simulink subsystem "Tractive_Motor_Ring_Single_Motor_subsys"  (R2020a)
settings: Solver=VariableStepAuto  StartTime=0.0  StopTime=10.0  RelTol=1e-3
undefined symbols (not defined in the file): DiscIntNeverNeededParam, magnitude, TMR
libraries: simulink x3
settings Model: Creator=Harjot  LastModifiedBy=Harjot

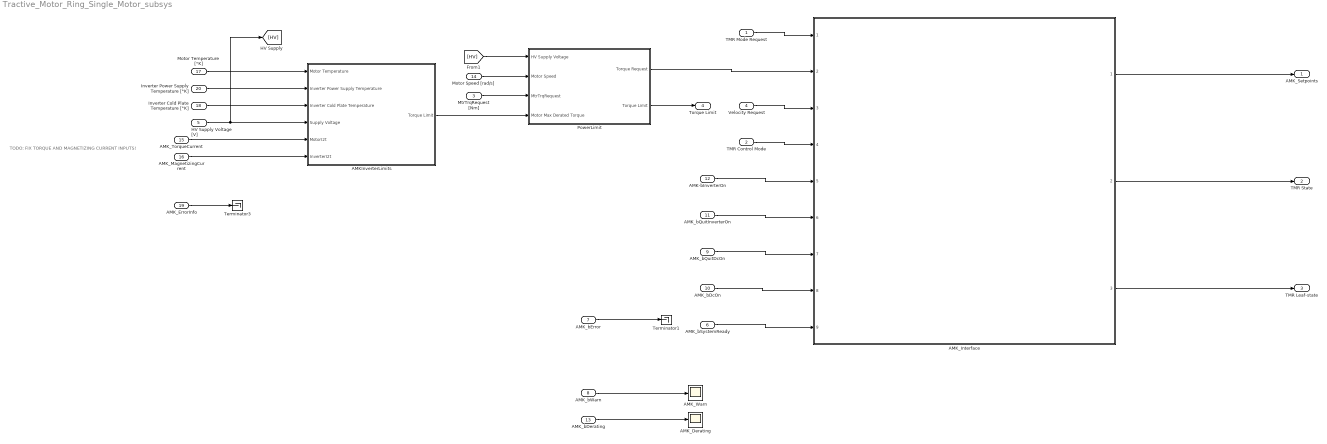
== system Tractive_Motor_Ring_Single_Motor_subsys ==
  note: TODO: FIX TORQUE AND MAGNETIZING CURRENT INPUTS!
  TMR Mode Request : Inport  RequirementInfo={} %GIDa_0b32f916_aa62_4ab6_a60b_804c209f055e
  TMR Control Mode : Inport  RequirementInfo={} %GIDa_899be42e_3bc9_4343_8c4c_9e024f0f1dcd  Port=2
  MtrTrqRequest [Nm] : Inport  RequirementInfo={} %GIDa_16bd7d4f_2c6d_4ce3_80ae_a158b09ca50a  Port=3
  Velocity Request : Inport  RequirementInfo={} %GIDa_36b15b8b_98d6_4bc3_9596_c4260eab6188  Port=4
  HV Supply Voltage [V] : Inport  RequirementInfo={} %GIDa_72d90ebf_0884_420f_b162_f30e0e78c23e  Port=5
  AMK_bSystemReady : Inport  RequirementInfo={} %GIDa_c8de1738_2ad1_42a2_b5d0_4f77bbb4223e  Port=6  OutDataTypeStr=boolean  Interpolate=off  LockScale=on
  AMK_bError : Inport  RequirementInfo={} %GIDa_a4d9bd43_86e5_45fc_8842_613fd797649f  Port=7  OutDataTypeStr=boolean  Interpolate=off  LockScale=on
  AMK_bWarn : Inport  RequirementInfo={} %GIDa_544a45c9_f4c4_4e73_8170_11e612af6fa1  Port=8  OutDataTypeStr=boolean  Interpolate=off
  AMK_bQuitDcOn : Inport  RequirementInfo={} %GIDa_da10d27a_d33e_4bd8_8507_d2659b32f1e7  Port=9  OutDataTypeStr=boolean  Interpolate=off  LockScale=on
  AMK_bDcOn : Inport  RequirementInfo={} %GIDa_1cca671d_68f3_48e8_91ed_5f6d9bdfc73e  Port=10  OutDataTypeStr=boolean  Interpolate=off  LockScale=on
  AMK_bQuitInverterOn : Inport  RequirementInfo={} %GIDa_2cbe62c1_b0a8_408a_a09b_cc028dfca1e6  Port=11  OutDataTypeStr=boolean  LockScale=on
  AMK-bInverterOn : Inport  RequirementInfo={} %GIDa_8fc59d25_5917_4f66_8f56_8f31af368e88  Port=12  OutDataTypeStr=boolean  Interpolate=off  LockScale=on
  AMK_bDerating : Inport  RequirementInfo={} %GIDa_fb751091_d4c7_4cff_997e_52806d3d30a0  Port=13  OutDataTypeStr=boolean  Interpolate=off
  Motor Speed [rad/s] : Inport  RequirementInfo={} %GIDa_f0ed834f_c372_4ce6_8264_ae369cf0457a  Port=14
  AMK_TorqueCurrent : Inport  RequirementInfo={} %GIDa_e0f8f9d2_51a7_4db7_9aed_c6e514902996  Port=15
  AMK_MagnetizingCurrent : Inport  RequirementInfo={} %GIDa_a3143f85_a5a8_4589_90ea_3cf1a5e0fe17  Port=16
  Motor Temperature [°K] : Inport  RequirementInfo={} %GIDa_e9626b0f_34d6_41dc_ba69_f3751265e366  Port=17  OutDataTypeStr=double
  Inverter Cold Plate Temperature [°K] : Inport  RequirementInfo={} %GIDa_17e3a5a5_9e9a_4c4f_a941_946527609ceb  Port=18  OutDataTypeStr=double
  AMK_ErrorInfo : Inport  RequirementInfo={} %GIDa_41130c06_a252_4499_9f77_2babee9d4883  Port=19  OutDataTypeStr=double
  Inverter Power Supply Temperature [°K] : Inport  RequirementInfo={} %GIDa_9e935b13_189d_44f7_8d48_34386f8f6a8c  Port=20  OutDataTypeStr=double
  AMKInverterLimits : Subsystem  RequirementInfo={} %GIDa_aa0f92cd_b864_4399_80e1_41da2508833f
  AMK_Derating : Scope
      settings: RequirementInfo={} %GIDa_4cc9d353_8262_40fa_bca2_02a298f34adf
  AMK_Interface : Subsystem  ReferencedSubsystem=AMK_Interface
  AMK_Warn : Scope
      settings: RequirementInfo={} %GIDa_434d5c32_d3ed_4195_97f3_de2a99eda9e5
  PowerLimit : Subsystem  RequirementInfo={} %GIDa_2476c70e_bf11_44e3_8c43_a3970cfd4237
  Terminator1 : Terminator
      settings: RequirementInfo={} %GIDa_851ef7c3_0e9b_48b0_a136_af49e9a5a281
  Terminator3 : Terminator
      settings: RequirementInfo={} %GIDa_67045959_67a9_4c05_97c7_ad8d9035b8be
  AMK_Setpoints : Outport  RequirementInfo={} %GIDa_22b8dc81_0cd3_4c20_ac91_ea8266b57b15  OutDataTypeStr=Bus: AmkSetpoints  VectorParamsAs1DForOutWhenUnconnected=off
  TMR State : Outport  RequirementInfo={} %GIDa_92497f2d_8924_487d_aba4_d0a8373c1186  Port=2  VectorParamsAs1DForOutWhenUnconnected=off
  TMR Leaf-state : Outport  RequirementInfo={} %GIDa_04fde0ce_78e9_4f67_91b5_da7d7284f00b  Port=3  VectorParamsAs1DForOutWhenUnconnected=off
  Torque Limit : Outport  RequirementInfo={} %GIDa_349136c5_bf5a_4487_833c_001109ddece7  Port=4  VectorParamsAs1DForOutWhenUnconnected=off
  wires:
  PowerLimit/2(Torque Limit) -> Torque Limit/1
  MtrTrqRequest [Nm]/1 -> PowerLimit/3(MtrTrqRequest)
  Motor Speed [rad/s]/1 -> PowerLimit/2(Motor Speed)
  AMKInverterLimits/1(Torque Limit) -> PowerLimit/4(Motor Max Derated Torque)
  AMK_bError/1 -> Terminator1/1
  [HV] -> PowerLimit/1(HV Supply Voltage)
  Inverter Power Supply Temperature [°K]/1 -> AMKInverterLimits/2(Inverter Power Supply Temperature)
  AMK_TorqueCurrent/1 -> AMKInverterLimits/5(MotorI2t)
  Inverter Cold Plate Temperature [°K]/1 -> AMKInverterLimits/3(Inverter Cold Plate Temperature)
  HV Supply Voltage [V]/1 -> [HV], AMKInverterLimits/4(Supply Voltage)
  AMK_MagnetizingCurrent/1 -> AMKInverterLimits/6(InverterI2t)
  AMK_Interface/1 -> AMK_Setpoints/1
  AMK_bDerating/1 -> AMK_Derating/1
  AMK_bWarn/1 -> AMK_Warn/1
  AMK_ErrorInfo/1 -> Terminator3/1
  Motor Temperature [°K]/1 -> AMKInverterLimits/1(Motor Temperature)
  TMR Mode Request/1 -> AMK_Interface/1
  PowerLimit/1(Torque Request) -> AMK_Interface/2
  Velocity Request/1 -> AMK_Interface/3
  TMR Control Mode/1 -> AMK_Interface/4
  AMK-bInverterOn/1 -> AMK_Interface/5
  AMK_bQuitInverterOn/1 -> AMK_Interface/6
  AMK_bQuitDcOn/1 -> AMK_Interface/7
  AMK_bDcOn/1 -> AMK_Interface/8
  AMK_bSystemReady/1 -> AMK_Interface/9
  AMK_Interface/2 -> TMR State/1
  AMK_Interface/3 -> TMR Leaf-state/1

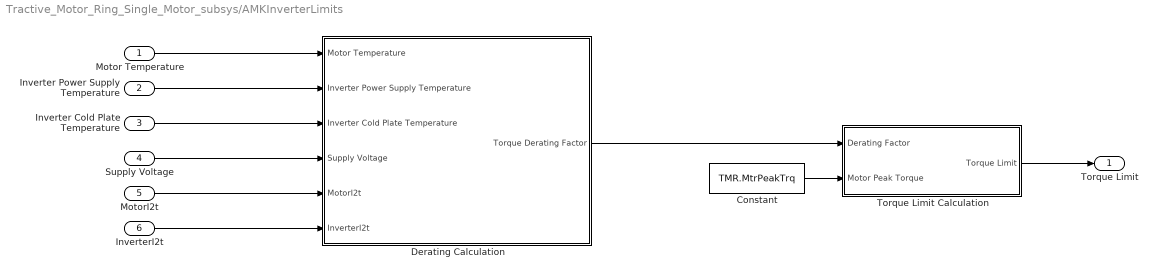
== system Tractive_Motor_Ring_Single_Motor_subsys/AMKInverterLimits ==
  Motor Temperature : Inport  RequirementInfo={} %GIDa_421d8d59_e97c_46c0_8684_f661b32e2da6
  Inverter Power Supply Temperature : Inport  RequirementInfo={} %GIDa_ea984ec6_eb38_4da7_bf5f_46f70598e9b8  Port=2
  Inverter Cold Plate Temperature : Inport  RequirementInfo={} %GIDa_a2f1bfb4_6059_4a9b_b9f6_b98a8575ec66  Port=3
  Supply Voltage : Inport  RequirementInfo={} %GIDa_b655bc3d_1fee_4859_9ee0_a3f0cc585127  Port=4
  MotorI2t : Inport  RequirementInfo={} %GIDa_d7a8d1db_e3d7_4d4e_8230_4144f8b06c4d  Port=5
  InverterI2t : Inport  RequirementInfo={} %GIDa_5c7a6706_2345_43d6_b9b7_ba06280ebe29  Port=6
  Constant : Constant  RequirementInfo={} %GIDa_a4805b7d_332c_4f8d_b926_1a627d2469f6  Value=TMR.MtrPeakTrq
  Derating Calculation : Subsystem  RequirementInfo={} %GIDa_5d32f30e_8689_4da7_9b84_9ed2f4df063a
  Torque Limit Calculation : Subsystem  RequirementInfo={} %GIDa_0c293d94_4945_4533_a0c2_e944d3e9cad5
  Torque Limit : Outport  RequirementInfo={} %GIDa_36fd4b23_a2c7_436c_a6a2_585403b7f1b4  VectorParamsAs1DForOutWhenUnconnected=off
  wires:
  Torque Limit Calculation/1(Torque Limit) -> Torque Limit/1
  InverterI2t/1 -> Derating Calculation/6(InverterI2t)
  Inverter Power Supply Temperature/1 -> Derating Calculation/2(Inverter Power Supply Temperature)
  Constant/1 -> Torque Limit Calculation/2(Motor Peak Torque)
  Motor Temperature/1 -> Derating Calculation/1(Motor Temperature)
  Derating Calculation/1(Torque Derating Factor) -> Torque Limit Calculation/1(Derating Factor)
  Inverter Cold Plate Temperature/1 -> Derating Calculation/3(Inverter Cold Plate Temperature)
  MotorI2t/1 -> Derating Calculation/5(MotorI2t)
  Supply Voltage/1 -> Derating Calculation/4(Supply Voltage)

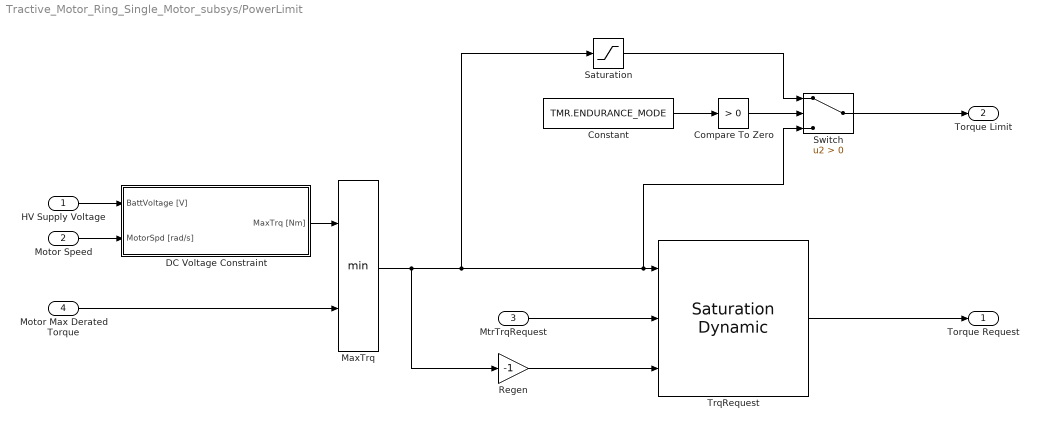
== system Tractive_Motor_Ring_Single_Motor_subsys/PowerLimit ==
  HV Supply Voltage : Inport  RequirementInfo={} %GIDa_c2e32798_cd4f_4c8a_a65a_728119494a4e
  Motor Speed : Inport  RequirementInfo={} %GIDa_933aee4b_e4b4_4104_a8a2_92c25e05beb2  Port=2
  MtrTrqRequest : Inport  RequirementInfo={} %GIDa_365dafb2_7a91_4d49_9a65_04040ec72de5  Port=3
  Motor Max Derated Torque : Inport  RequirementInfo={} %GIDa_7f63b285_d843_4e70_9e32_221f08d053be  Port=4
  Compare To Zero : simulink/Logic and Bit Operations/Compare To Zero  RequirementInfo={} %GIDa_c9d13251_2199_4b8b_aa35_020b89726b08  relop=>  OutDataTypeStr=boolean
  Constant : Constant  RequirementInfo={} %GIDa_5dbf2ca4_cbeb_44aa_b8ec_92adadf3a31c  Value=TMR.ENDURANCE_MODE
  DC Voltage Constraint : Subsystem  RequirementInfo={} %GIDa_92c81348_b4c9_40da_9741_e1962b84860f
  MaxTrq : MinMax  RequirementInfo={} %GIDa_1818b7d5_8d0e_4b0e_90fc_eee558479f24  Inputs=2
  Regen : Gain  RequirementInfo={} %GIDa_c9b8d0fc_8531_4bac_897a_2c2ec2a6688d  Gain=-1
  Saturation : Saturate  RequirementInfo={} %GIDa_8ddb1a86_ed92_4c81_9452_61601b67b037  UpperLimit=TMR.MtrNominalTrq  LowerLimit=0
  Switch : Switch  RequirementInfo={} %GIDa_99d8f9f2_d0f3_489c_94e7_4d69a13899fd  Criteria=u2 > Threshold
  TrqRequest : simulink/Discontinuities/Saturation Dynamic  RequirementInfo={} %GIDa_8252a3f5_2b8a_431a_b628_5b81ae0f8fad  OutMin=[]  OutMax=[]  OutDataTypeStr=Inherit: Same as second input  OutDataType=fixdt(1, 16)  OutScaling=2^-10  DoSatur=off
  Torque Request : Outport  RequirementInfo={} %GIDa_a697b8a4_e6b0_40d7_a2f6_8a132d380153  VectorParamsAs1DForOutWhenUnconnected=off
  Torque Limit : Outport  RequirementInfo={} %GIDa_9cb23760_879e_4fdb_85f6_377f72198434  Port=2  VectorParamsAs1DForOutWhenUnconnected=off
  wires:
  Saturation/1 -> Switch/1
  Switch/1 -> Torque Limit/1
  Compare To Zero/1 -> Switch/2
  Constant/1 -> Compare To Zero/1
  Regen/1 -> TrqRequest/3
  HV Supply Voltage/1 -> DC Voltage Constraint/1(BattVoltage [V])
  DC Voltage Constraint/1(MaxTrq [Nm]) -> MaxTrq/1
  MaxTrq/1 -> TrqRequest/1, Switch/3, Saturation/1, Regen/1
  Motor Speed/1 -> DC Voltage Constraint/2(MotorSpd [rad/s])
  TrqRequest/1 -> Torque Request/1
  Motor Max Derated Torque/1 -> MaxTrq/2
  MtrTrqRequest/1 -> TrqRequest/2

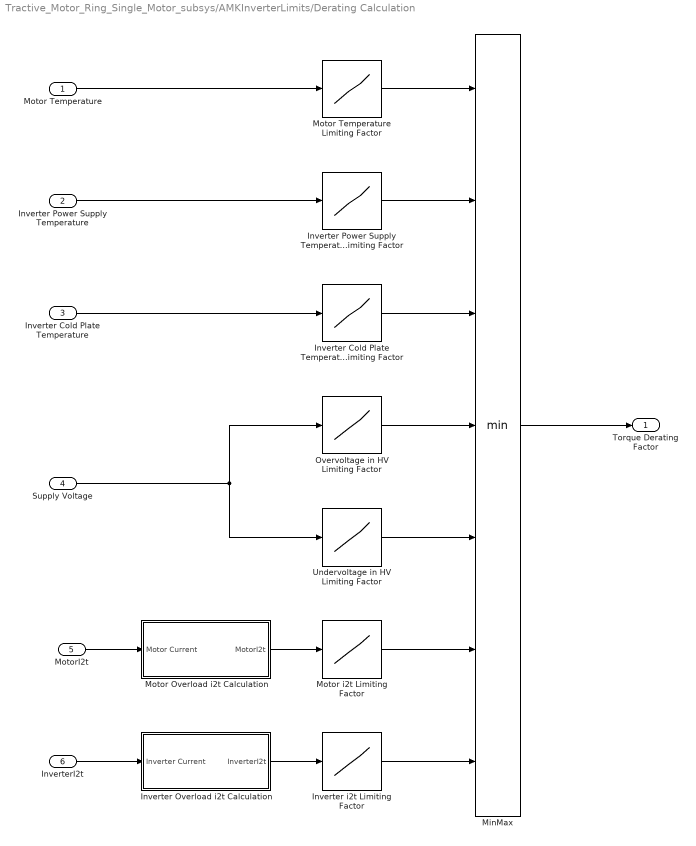
== system Tractive_Motor_Ring_Single_Motor_subsys/AMKInverterLimits/Derating Calculation ==
  Motor Temperature : Inport  RequirementInfo={} %GIDa_204401dd_a26d_4c4a_a9ed_9ebd30f16e89
  Inverter Power Supply Temperature : Inport  RequirementInfo={} %GIDa_f4617428_dec0_47a8_91e6_d3677d00ce52  Port=2
  Inverter Cold Plate Temperature : Inport  RequirementInfo={} %GIDa_9ebdb56a_af85_4a5e_bd69_6c13f7b23dcb  Port=3
  Supply Voltage : Inport  RequirementInfo={} %GIDa_4a971c51_909b_4e2f_9e5d_2c8b9170f21d  Port=4
  MotorI2t : Inport  RequirementInfo={} %GIDa_878f7ac8_46c5_4716_98cf_a1a4baabae38  Port=5
  InverterI2t : Inport  RequirementInfo={} %GIDa_77b82b5e_623a_4612_831c_fa1e833f1d16  Port=6
  Inverter Cold Plate Temperature Limiting Factor : Lookup_n-D  RequirementInfo={} %GIDa_7a3ea9b9_c29f_4161_95be_c382916e9550  NumberOfTableDimensions=1  BreakpointsForDimension1=[TMR.ColdPlateTempFullTrq, TMR.ColdPlateTempNoTrq]  Table=[1,0]  ExtrapMethod=Clip  InternalRulePriority=Speed  RndMeth=Simplest  InputSameDT=on
  Inverter Overload i2t Calculation : Subsystem  RequirementInfo={} %GIDa_3441df8e_d71d_4c27_964f_79081b2c843f
  Inverter Power Supply Temperature Limiting Factor : Lookup_n-D  RequirementInfo={} %GIDa_fb230598_dfe0_42b9_ac80_b67de67f7b74  NumberOfTableDimensions=1  BreakpointsForDimension1=[TMR.PwrSpplyTempFullTrq, TMR.PwrSpplyTempNoTrq]  Table=[1,0]  ExtrapMethod=Clip  InternalRulePriority=Speed  RndMeth=Simplest  InputSameDT=on
  Inverter i2t Limiting Factor : Lookup_n-D  RequirementInfo={} %GIDa_f3f4ec3a_3c41_4fff_bb42_91f9abcc7cf7  NumberOfTableDimensions=1  BreakpointsForDimension1=[TMR.InvCurrOverloadThreshold*TMR.InvI2t, TMR.InvI2t]  Table=[1,0]  ExtrapMethod=Clip  InternalRulePriority=Speed  RndMeth=Simplest  InputSameDT=on
  MinMax : MinMax  RequirementInfo={} %GIDa_c5589417_6b99_479b_bbab_952416d8dd64  Inputs=7
  Motor Overload i2t Calculation : Subsystem  RequirementInfo={} %GIDa_6bcc5a01_e28b_4b16_8331_2fcd4d12553f
  Motor Temperature Limiting Factor : Lookup_n-D  RequirementInfo={} %GIDa_fcbe106c_3c49_4470_aa70_4372ccef9a91  NumberOfTableDimensions=1  BreakpointsForDimension1=[TMR.MtrTempFullTrq, TMR.MtrTempNoTrq]  Table=[1,0]  ExtrapMethod=Clip  InternalRulePriority=Speed  RndMeth=Simplest  InputSameDT=on
  Motor i2t Limiting Factor : Lookup_n-D  RequirementInfo={} %GIDa_64a6c4dc_a943_4623_9ac2_7ff1559e1b08  NumberOfTableDimensions=1  BreakpointsForDimension1="[TMR.MtrCurrOverloadThreshold*TMR.MtrI2t,  TMR.MtrI2t]"  Table=[1,0]  ExtrapMethod=Clip  InternalRulePriority=Speed  RndMeth=Simplest  InputSameDT=on
  Overvoltage in HV Limiting Factor : Lookup_n-D  RequirementInfo={} %GIDa_bf9ca155_9e06_42ac_bda7_11ac6a5b2543  NumberOfTableDimensions=1  BreakpointsForDimension1=[TMR.HighBatteryVolt, TMR.MaxBatteryVolt]  Table=[1,0]  ExtrapMethod=Clip  InternalRulePriority=Speed  RndMeth=Simplest  InputSameDT=on
  Undervoltage in HV Limiting Factor : Lookup_n-D  RequirementInfo={} %GIDa_f9167007_5e7d_4824_a668_e705c7865b04  NumberOfTableDimensions=1  BreakpointsForDimension1=[TMR.MinBatteryVolt, TMR.LowBatteryVolt]  Table=[0,1]  ExtrapMethod=Clip  InternalRulePriority=Speed  RndMeth=Simplest  InputSameDT=on
  Torque Derating Factor : Outport  RequirementInfo={} %GIDa_4ab78645_0b52_462e_bf14_5e5a6c6b9afe  VectorParamsAs1DForOutWhenUnconnected=off
  wires:
  Motor i2t Limiting Factor/1 -> MinMax/6
  Inverter i2t Limiting Factor/1 -> MinMax/7
  InverterI2t/1 -> Inverter Overload i2t Calculation/1(Inverter Current)
  Undervoltage in HV Limiting Factor/1 -> MinMax/5
  Inverter Power Supply Temperature Limiting Factor/1 -> MinMax/2
  Motor Temperature Limiting Factor/1 -> MinMax/1
  Overvoltage in HV Limiting Factor/1 -> MinMax/4
  Motor Temperature/1 -> Motor Temperature Limiting Factor/1
  Inverter Cold Plate Temperature Limiting Factor/1 -> MinMax/3
  Inverter Cold Plate Temperature/1 -> Inverter Cold Plate Temperature Limiting Factor/1
  Inverter Power Supply Temperature/1 -> Inverter Power Supply Temperature Limiting Factor/1
  MotorI2t/1 -> Motor Overload i2t Calculation/1(Motor Current)
  Motor Overload i2t Calculation/1(MotorI2t) -> Motor i2t Limiting Factor/1
  Supply Voltage/1 -> Undervoltage in HV Limiting Factor/1, Overvoltage in HV Limiting Factor/1
  Inverter Overload i2t Calculation/1(InverterI2t) -> Inverter i2t Limiting Factor/1
  MinMax/1 -> Torque Derating Factor/1

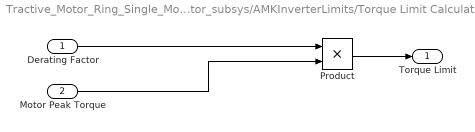
== system Tractive_Motor_Ring_Single_Motor_subsys/AMKInverterLimits/Torque Limit Calculation ==
  Derating Factor : Inport  RequirementInfo={} %GIDa_fd6b3c22_f3af_456e_ab14_995e66b71a6e
  Motor Peak Torque : Inport  RequirementInfo={} %GIDa_c93655c4_a015_4261_b947_2f749186f374  Port=2
  Product : Product  RequirementInfo={} %GIDa_abb5b4e5_d2ff_4e1f_a21e_60e0bca55249
  Torque Limit : Outport  RequirementInfo={} %GIDa_6ffda1d4_6d5a_4d8a_a06b_08b6a2d0be15  VectorParamsAs1DForOutWhenUnconnected=off
  wires:
  Product/1 -> Torque Limit/1
  Derating Factor/1 -> Product/1
  Motor Peak Torque/1 -> Product/2

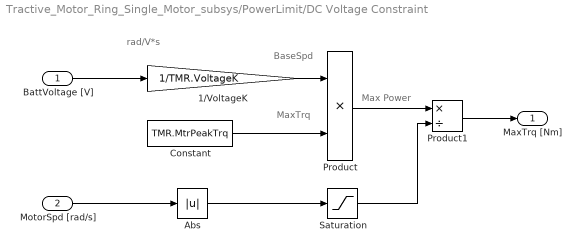
== system Tractive_Motor_Ring_Single_Motor_subsys/PowerLimit/DC Voltage Constraint ==
  note: Max Power
  note: MaxTrq
  note: BaseSpd
  note: rad/V*s
  BattVoltage [V] : Inport  RequirementInfo={} %GIDa_d70c9c14_ae20_449f_95f5_51e60b3e27cd
  MotorSpd [rad/s] : Inport  RequirementInfo={} %GIDa_4b490560_2eac_4941_bf79_d455b8a22d89  Port=2
  1/VoltageK : Gain  RequirementInfo={} %GIDa_5b9d2ba3_5723_43d0_9685_958bee8e36d4  Gain=1/TMR.VoltageK
  Abs : Abs  RequirementInfo={} %GIDa_cff544dd_3732_43b4_ad98_2a5702883f73
  Constant : Constant  RequirementInfo={} %GIDa_6ec80ac5_5d41_4f57_a81d_228a62a29840  Value=TMR.MtrPeakTrq
  Product : Product  RequirementInfo={} %GIDa_2e9569d8_c03a_4bc1_a9a2_48e5241925d0
  Product1 : Product  RequirementInfo={} %GIDa_8083fe5f_8c89_4253_a32e_904dfae0a255  Inputs=*/
  Saturation : Saturate  RequirementInfo={} %GIDa_3cb079c8_13fa_4bcf_a92d_0a3ca5223395  UpperLimit=10000  LowerLimit=TMR.MinMtrSpd
  MaxTrq [Nm] : Outport  RequirementInfo={} %GIDa_2802e1ae_2c30_460b_907c_8084c4e9cf48  VectorParamsAs1DForOutWhenUnconnected=off
  wires:
  Saturation/1 -> Product1/2
  Product/1 -> Product1/1
  BattVoltage [V]/1 -> 1/VoltageK/1
  Constant/1 -> Product/2
  Product1/1 -> MaxTrq [Nm]/1
  MotorSpd [rad/s]/1 -> Abs/1
  1/VoltageK/1 -> Product/1
  Abs/1 -> Saturation/1

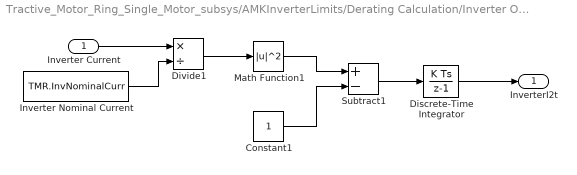
== system Tractive_Motor_Ring_Single_Motor_subsys/AMKInverterLimits/Derating Calculation/Inverter Overload i2t Calculation ==
  Inverter Current : Inport  RequirementInfo={} %GIDa_0f345d63_277d_4471_a466_c89ac27940e7
  Constant1 : Constant  RequirementInfo={} %GIDa_a27e5077_5bc0_4742_89d4_8f0e233f992d
  Discrete-Time Integrator : DiscreteIntegrator  RequirementInfo={} %GIDa_90e65162_d51b_4c08_a29e_7d9e074ad865  SampleTime=-1  ICPrevOutput=DiscIntNeverNeededParam  ICPrevScaledInput=DiscIntNeverNeededParam
  Divide1 : Product  RequirementInfo={} %GIDa_dcb640f9_8d83_4d0a_b852_c9ce71f16fd7  Inputs=*/
  Inverter Nominal Current : Constant  RequirementInfo={} %GIDa_80c6a464_ec3e_44d3_a78b_ea4efa55c4b7  Value=TMR.InvNominalCurr
  Math Function1 : Math  RequirementInfo={} %GIDa_08805274_6108_4951_a7f1_3d505fcdc46f  Operator=magnitude^2  SignedPower=on  SaturateOnIntegerOverflow=on
  Subtract1 : Sum  RequirementInfo={} %GIDa_6f58b2ea_9d45_44a4_ab59_aafca238619d  Inputs=+-
  InverterI2t : Outport  RequirementInfo={} %GIDa_fbf7ef9e_1cf5_4baf_9b2d_71d3dc0d780f  VectorParamsAs1DForOutWhenUnconnected=off
  wires:
  Subtract1/1 -> Discrete-Time Integrator/1
  Constant1/1 -> Subtract1/2
  Inverter Nominal Current/1 -> Divide1/2
  Discrete-Time Integrator/1 -> InverterI2t/1
  Inverter Current/1 -> Divide1/1
  Divide1/1 -> Math Function1/1
  Math Function1/1 -> Subtract1/1

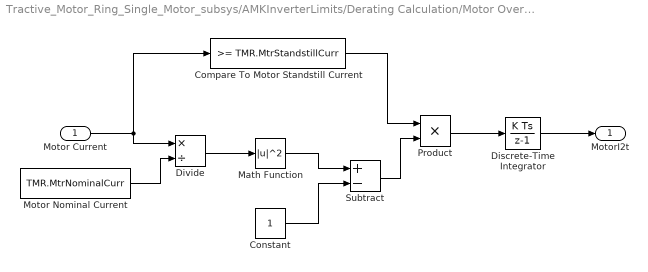
== system Tractive_Motor_Ring_Single_Motor_subsys/AMKInverterLimits/Derating Calculation/Motor Overload i2t Calculation ==
  Motor Current : Inport  RequirementInfo={} %GIDa_086af66c_bacf_4523_aa39_c4ae0452038e
  Compare To Motor Standstill Current : simulink/Logic and Bit Operations/Compare To Constant  RequirementInfo={} %GIDa_8128cf5b_a349_4347_9996_6df328df5b87  relop=>=  const=TMR.MtrStandstillCurr  OutDataTypeStr=boolean
  Constant : Constant  RequirementInfo={} %GIDa_08fcf0ae_049e_41a1_b457_d804b1245447
  Discrete-Time Integrator : DiscreteIntegrator  RequirementInfo={} %GIDa_cd69074b_64ca_43eb_9536_4ba718159bf0  SampleTime=-1  ICPrevOutput=DiscIntNeverNeededParam  ICPrevScaledInput=DiscIntNeverNeededParam
  Divide : Product  RequirementInfo={} %GIDa_9cd1e926_6e59_45cc_8df3_15ed29d03ea3  Inputs=*/
  Math Function : Math  RequirementInfo={} %GIDa_b4acf5a4_85ac_4f9e_bb84_33e7c9c60d50  Operator=magnitude^2  SignedPower=on  SaturateOnIntegerOverflow=on
  Motor Nominal Current : Constant  RequirementInfo={} %GIDa_955ba5f8_d8c0_4e23_b5e8_8ce81bd7e852  Value=TMR.MtrNominalCurr
  Product : Product  RequirementInfo={} %GIDa_1ef4a749_4dd9_4af6_aec3_2d5d8945c4a1
  Subtract : Sum  RequirementInfo={} %GIDa_8619936b_41a9_4772_a2f9_beac25f02cf5  Inputs=+-
  MotorI2t : Outport  RequirementInfo={} %GIDa_8decadf0_ddf5_4b3a_9e49_6ea0aa67dbb4  VectorParamsAs1DForOutWhenUnconnected=off
  wires:
  Motor Current/1 -> Divide/1, Compare To Motor Standstill Current/1
  Divide/1 -> Math Function/1
  Math Function/1 -> Subtract/1
  Subtract/1 -> Product/2
  Compare To Motor Standstill Current/1 -> Product/1
  Motor Nominal Current/1 -> Divide/2
  Product/1 -> Discrete-Time Integrator/1
  Constant/1 -> Subtract/2
  Discrete-Time Integrator/1 -> MotorI2t/1
